simulink model "hexacopter_sim"  (R2023a)
settings: Solver=VariableStepAuto  StartTime=0.0  StopTime=15  MaxStep=0.001  RelTol=1e-7  EnableMultiTasking=on
values from neighbouring files (symbols this model uses):
  arm_length = 0.35    [hexacopter.m]    (also in hexacopter_unmodified.m)
  batteryDistanceFromCOG = -0.1    [hexacopter.m]    (also in hexacopter_unmodified.m)
  batteryMass = 0.56*2    (= 1.12)    [hexacopter.m]    (also in hexacopter_unmodified.m)
  batVolt = 3.7*cells    (= 14.8)    [hexacopter.m]    (also in hexacopter_unmodified.m)
  bodyMass = 1.2    [hexacopter.m]    (also in hexacopter_unmodified.m)
  deadCurrent = 0.3    [hexacopter.m]    (also in hexacopter_unmodified.m)
  droneMass = bodyMass + motorCount*(motorMass + propellerMassRaw)    (= 2.424)    [hexacopter.m]    (also in hexacopter_unmodified.m)
  h1al = 0.07    [discrete_controller_tuning.m]    (also in height_controller.m; hexacopter.m; hexacopter_unmodified.m)
  h1kp = 60    [hexacopter.m]    (also in hexacopter_unmodified.m)
  h1td = 1 / (sqrt(h1al) * target)    [height_controller.m]    (also in hexacopter.m = 1; hexacopter_unmodified.m = 1)
  h1ti = h1Ni * (1/ target)    (= 1.27118644068)    [height_controller.m]    (also in hexacopter.m = 1; hexacopter_unmodified.m = 1)
  h1val = 0.6    [discrete_controller_tuning.m]    (also in hexacopter.m = 0)
  h1vkp = 1    [hexacopter.m]
  h1vtd = 0    [hexacopter.m]
  h1vti = 1    [hexacopter.m]
  h_beta = 5    [hexacopter.m]    (also in hexacopter_unmodified.m)
  h_tau = 1.5    [hexacopter.m]    (also in hexacopter_unmodified.m)
  hoverControl = hoverVoltage/batVolt*1024    [hexacopter.m]    (also in hexacopter_unmodified.m)
  hoverVoltage = hoverCurrent * Ra + hoverRPM / Kv    [hexacopter.m]    (also in hexacopter_unmodified.m)
  KDrag = 1.5e-9    (= 1.5e-09)    [hexacopter.m]    (also in hexacopter_unmodified.m)
  Km = 60/(Kv * 2 * pi)    (= 0.013641852265)    [hexacopter.m]    (also in hexacopter_unmodified.m)
  Ktrust = 2.7e-5    (= 2.7e-05)    [hexacopter.m]    (also in hexacopter_unmodified.m)
  minimumMotorVolt = 1.0    (= 1)    [hexacopter.m]    (also in hexacopter_unmodified.m)
  motorMass = motorOnlyMass + 0.085    (= 0.187)    [hexacopter.m]    (also in hexacopter_unmodified.m)
  N = solve(eqn,V)    [temp.m]
  paal = 0.2    [hexacopter.m]    (also in hexacopter_unmodified.m)
  pakp = 0    [hexacopter.m]    (also in hexacopter_unmodified.m)
  pal = 0.5    [hexacopter.m]    (also in hexacopter_unmodified.m)
  patd = 1    [hexacopter.m]    (also in hexacopter_unmodified.m)
  pati = 100    [hexacopter.m]    (also in hexacopter_unmodified.m)
  pkp = 0    [hexacopter.m]    (also in hexacopter_unmodified.m)
  propellerMass = propellerMassRaw + 3*motorInertia/propellerRadius^2    (= 0.0220980494455)    [hexacopter.m]    (also in hexacopter_unmodified.m)
  ptd = 1    [hexacopter.m]    (also in hexacopter_unmodified.m)
  pti = 1    [hexacopter.m]    (also in hexacopter_unmodified.m)
  pushEnabled = 0    [hexacopter.m]    (also in hexacopter_unmodified.m)
  Ra = 0.083    [hexacopter.m]    (also in hexacopter_unmodified.m)
  raal = 0.2    [hexacopter.m]    (also in hexacopter_unmodified.m)
  rakp = 0    [hexacopter.m]    (also in hexacopter_unmodified.m)
  ral = 0.5    [hexacopter.m]    (also in hexacopter_unmodified.m)
  ratd = 1    [hexacopter.m]    (also in hexacopter_unmodified.m)
  rati = 100    [hexacopter.m]    (also in hexacopter_unmodified.m)
  rkp = 0    [hexacopter.m]    (also in hexacopter_unmodified.m)
  roll_limit = 10    [hexacopter.m]    (also in hexacopter_unmodified.m)
  rtd = 1    [hexacopter.m]    (also in hexacopter_unmodified.m)
  rti = 1    [hexacopter.m]    (also in hexacopter_unmodified.m)
  xal = 0.2    [hexacopter.m]    (also in hexacopter_unmodified.m = 1)
  xkp = 0    [hexacopter.m]    (also in hexacopter_unmodified.m)
  xtd = 1    [hexacopter.m]    (also in hexacopter_unmodified.m)
  xti = 100    [hexacopter.m]    (also in hexacopter_unmodified.m)
  xval = 0.2    [hexacopter.m]    (also in hexacopter_unmodified.m = 0.3; vel_controller.m = 0.3)
  xvkp = 0    [hexacopter.m]    (also in hexacopter_unmodified.m; vel_controller.m = 0.184077200147)
  xvtd = 1    [hexacopter.m]    (also in hexacopter_unmodified.m; vel_controller.m = 1 / (sqrt(xval) * target))
  xvti = 100    [hexacopter.m]    (also in hexacopter_unmodified.m; vel_controller.m = 0)
  yaal = 0.5    [hexacopter.m]    (also in hexacopter_unmodified.m)
  yakp = 0    [hexacopter.m]    (also in hexacopter_unmodified.m)
  yal = 0.5    [hexacopter.m]    (also in hexacopter_unmodified.m)
  yatd = 1    [hexacopter.m]    (also in hexacopter_unmodified.m)
  yati = 100    [hexacopter.m]    (also in hexacopter_unmodified.m)
  yaw_limit = 45    [hexacopter.m]    (also in hexacopter_unmodified.m)
  yiLim = 500    [hexacopter.m]    (also in hexacopter_unmodified.m)
  ykp = 0    [hexacopter.m]    (also in hexacopter_unmodified.m)
  ytd = 0    [hexacopter.m]    (also in hexacopter_unmodified.m)
  yti = 1000    [hexacopter.m]    (also in hexacopter_unmodified.m)
  yval = 0.3    [hexacopter.m]    (also in hexacopter_unmodified.m)
  yvkp = 0    [hexacopter.m]    (also in hexacopter_unmodified.m)
  yvtd = 1    [hexacopter.m]    (also in hexacopter_unmodified.m)
  yvti = 100    [hexacopter.m]    (also in hexacopter_unmodified.m)
undefined symbols (not defined in the file or in its folder): h2al, h2kp, h2td, h2ti, X, Y, Z
libraries: sm_lib x52, nesl_utility x34, simulink x3
(part 1 of 3)
settings Model: Creator=chr  LastModifiedBy=marcu
settings SolverCC: AlgebraicLoopSolver=TrustRegion
settings DataIOCC: LimitDataPoints=on  SaveFormat=Array  ReturnWorkspaceOutputs=off
settings OptimizationCC: LifeSpan=inf
settings DebuggingCC: UnconnectedInputMsg=warning  UnconnectedOutputMsg=warning  UnconnectedLineMsg=warning  SFUnexpectedBacktrackingDiag=warning  SFNoUnconditionalDefaultTransitionDiag=warning  SFExecutionAtInitializationDiag=none  ArithmeticOperatorsInVariantConditions=warning
settings HardwareCC: ProdBitPerPointer=32  ProdBitPerSizeT=32  ProdBitPerPtrDiffT=32  ProdLargestAtomicFloat=None  ProdIntDivRoundTo=Undefined  ProdEndianess=Unspecified  ProdWordSize=32  ProdHWDeviceType=32-bit Generic
settings ModelReferenceCC: EnableRefExpFcnMdlSchedulingChecks=on  PropagateSignalLabelsOutOfModel=off
settings SFSimCC: SimUseLocalCustomCode=off  CustomCodeUndefinedFunction=UseInterfaceOnly
settings RTWCC: RTWUseLocalCustomCode=off  DLArmComputeVersion=19.05
settings CodeAppCC: StateflowObjectComments=on
settings GRTTargetCC: TargetLangStandard=C89/C90 (ANSI)
settings ConfigComp: CovMetricSettings=dw  CovSaveCumulativeToWorkspaceVar=on  CovSaveSingleToWorkspaceVar=on  CovExternalEMLEnable=off
settings SimscapeCC: SimscapeNormalizeSystem=off  SimscapeLogType=all  SimscapeLogDataHistory=10000
settings ConfigurationSet: Description=SimMechanics 2G

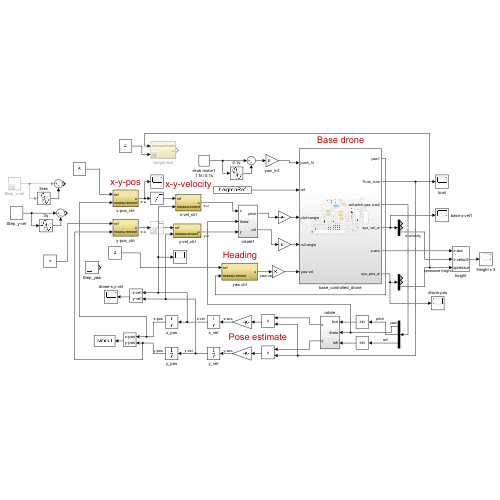
[thumbnail: Simulink's stored preview of the top-level diagram]
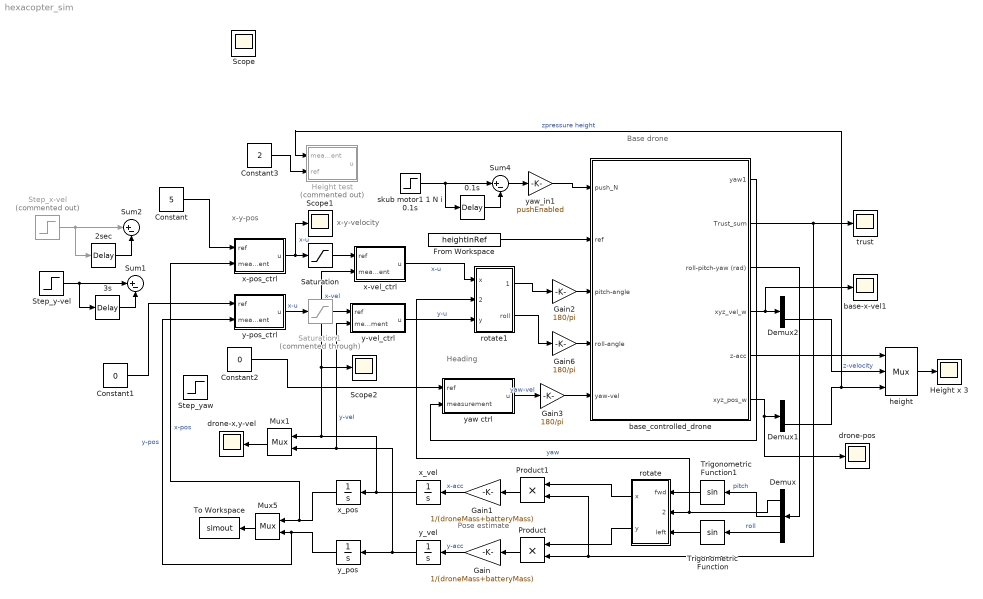
== system hexacopter_sim ==
  note: x-y-velocity
  note: Heading
  note: Pose estimate
  note: Base drone
  note: x-y-pos
  0.1s : TransportDelay  DelayTime=0.1
  2sec : TransportDelay  DelayTime=2
  3s : TransportDelay  DelayTime=2
  Constant : Constant  Value=5
  Constant1 : Constant  Value=0
  Constant2 : Constant  Value=0
  Constant3 : Constant  Value=2
  Demux : Demux  Outputs=3
  Demux1 : Demux  Outputs=3
  Demux2 : Demux  Outputs=3
  From Workspace : FromWorkspace  VariableName=heightInRef
  Gain : Gain  Gain=1/(droneMass+batteryMass)
  Gain1 : Gain  Gain=1/(droneMass+batteryMass)
  Gain2 : Gain  Gain=180/pi
  Gain3 : Gain  Gain=180/pi
  Gain6 : Gain  Gain=180/pi
  Height test : Subsystem  Commented=on
  Height x 3 : Scope
  Mux1 : Mux  Inputs=2
      settings: DisplayOption=signals
  Mux5 : Mux  Inputs=2
      settings: DisplayOption=signals
  Product : Product
  Product1 : Product
  Saturation : Saturate  UpperLimit=1  LowerLimit=-1
  Saturation1 : Saturate  Commented=through  UpperLimit=1  LowerLimit=-1
  Scope1 : Scope
  Scope2 : Scope
  Step_x-vel : Step  Commented=on  Time=5  After=0.1  SampleTime=0
  Step_y-vel : Step  Time=3  After=4  SampleTime=0
  Step_yaw : Step  Time=3.0  After=pi/2  SampleTime=0
  Sum1 : Sum  Inputs=|+-
  Sum2 : Sum  Inputs=|+-
  Sum4 : Sum  Inputs=|+-
  To Workspace : ToWorkspace  VariableName=simout  SaveFormat=Timeseries  SampleTime=-1
  Trigonometric Function : Trigonometry
  Trigonometric Function1 : Trigonometry
  base-x-vel1 : Scope
  base_controlled_drone : Subsystem
  drone-pos : Scope
  drone-x,y-vel : Scope
  height : Mux  Inputs=3
      settings: DisplayOption=signals
  rotate : Subsystem
  rotate1 : Subsystem
  skub motor1 1 N i 0.1s : Step  Time=2  After=4  SampleTime=0
  trust : Scope
  x-pos_ctrl : Subsystem
  x-vel_ctrl : Subsystem
  x_pos : Integrator
  x_vel : Integrator
  y-pos_ctrl : Subsystem
  y-vel_ctrl : Subsystem
  y_pos : Integrator
  y_vel : Integrator
  yaw ctrl : Subsystem
  yaw_in1 : Gain  Gain=pushEnabled
  Scope : Scope
  wires:
  Product/1 -> Gain/1
  Gain/1 -> y_vel/1  "y-acc"
  y_vel/1 -> y_pos/1, Mux1/2, y-vel_ctrl/2(measurement)  "y-vel"
  x_vel/1 -> x_pos/1, Mux1/1, x-vel_ctrl/2(measurement), Scope2/1  "x-vel"
  Gain1/1 -> x_vel/1  "x-acc"
  Product1/1 -> Gain1/1
  Mux1/1 -> drone-x,y-vel/1
  Mux5/1 -> To Workspace/1
  x_pos/1 -> x-pos_ctrl/2(measurement), Mux5/1  "x-pos"
  y_pos/1 -> y-pos_ctrl/2(measurement), Mux5/2  "y-pos"
  base_controlled_drone/5(z-acc) -> height/1
  base_controlled_drone/2(Trust_sum) -> trust/1, Product1/2, Product/2
  Demux1/3 -> Height test/1(measurement), height/3  "zpressure height"
  yaw ctrl/1(u) -> Gain3/1  "yaw-vel"
  base_controlled_drone/1(yaw1) -> yaw ctrl/2(measurement)
  base_controlled_drone/3(roll-pitch-yaw (rad)) -> Demux/1
  base_controlled_drone/4(xyz_vel_w) -> base-x-vel1/1, Demux2/1
  base_controlled_drone/6(xyz_pos_w) -> Demux1/1, drone-pos/1
  Demux2/3 -> height/2  "z-velocity"
  Demux/3 -> Trigonometric Function/1  "roll"
  Demux/2 -> Trigonometric Function1/1  "pitch"
  0.1s/1 -> Sum4/2
  skub motor1 1 N i 0.1s/1 -> 0.1s/1, Sum4/1
  Sum4/1 -> yaw_in1/1
  yaw_in1/1 -> base_controlled_drone/1(push_N)
  Step_y-vel/1 -> 3s/1, Sum1/1
  3s/1 -> Sum1/2
  2sec/1 -> Sum2/2
  Step_x-vel/1 -> 2sec/1, Sum2/1
  y-vel_ctrl/1(u) -> rotate1/3(y)  "y-u"
  Trigonometric Function1/1 -> rotate/1(fwd)
  Demux/1 -> rotate1/2(theta), rotate/2(theta)  "yaw"
  Trigonometric Function/1 -> rotate/3(left)
  rotate/1(x) -> Product1/1
  rotate/2(y) -> Product/1
  x-vel_ctrl/1(u) -> rotate1/1(x)  "x-u"
  rotate1/1(pitch) -> Gain2/1
  rotate1/2(roll) -> Gain6/1
  Gain6/1 -> base_controlled_drone/4(roll-angle)
  Gain2/1 -> base_controlled_drone/3(pitch-angle)
  Gain3/1 -> base_controlled_drone/5(yaw-vel)
  Constant1/1 -> y-pos_ctrl/1(ref)
  Constant/1 -> x-pos_ctrl/1(ref)
  x-pos_ctrl/1(u) -> Scope1/1, Saturation/1  "x-u"
  y-pos_ctrl/1(u) -> Saturation1/1  "x-u"
  Constant2/1 -> yaw ctrl/1(ref)
  Constant3/1 -> Height test/2(ref)
  Saturation1/1 -> y-vel_ctrl/1(ref)
  Saturation/1 -> x-vel_ctrl/1(ref)
  From Workspace/1 -> base_controlled_drone/2(ref)
  height/1 -> Height x 3/1

== system hexacopter_sim/Height test ==
  measurement : Inport
  ref : Inport  Port=2
  Constant : Constant  Value=hoverControl
  Gain : Gain  Gain=h2kp
  Gain1 : Gain  Gain=1/h2ti
  Gain2 : Gain  Gain=1/102.4
  Integrator : Integrator  InitialCondition=hoverVoltage  LimitOutput=on  UpperSaturationLimit=batVolt  LowerSaturationLimit=-batVolt
  Sum : Sum  Inputs=|+-
  Sum1 : Sum  Inputs=+++
  Transfer Fcn : TransferFcn  Numerator=[h2td 1]  Denominator=[h2al*h2td 1]
  u : Outport  VectorParamsAs1DForOutWhenUnconnected=off
  wires:
  ref/1 -> Sum/1
  measurement/1 -> Transfer Fcn/1
  Transfer Fcn/1 -> Sum/2
  Sum/1 -> Gain/1
  Integrator/1 -> Sum1/2
  Gain/1 -> Sum1/3, Gain1/1
  Gain1/1 -> Integrator/1
  Sum1/1 -> u/1
  Constant/1 -> Gain2/1
  Gain2/1 -> Sum1/1

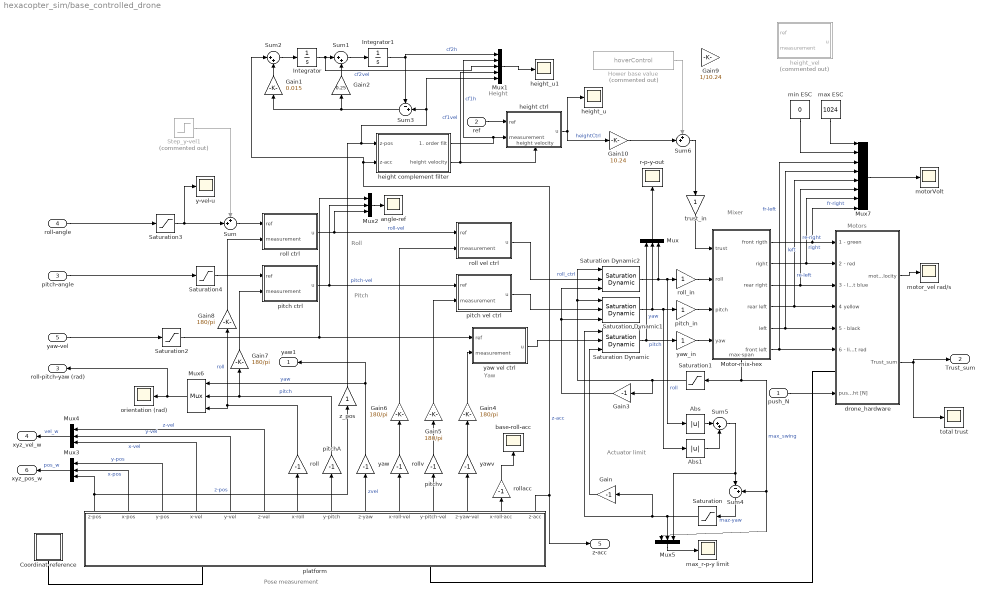
== system hexacopter_sim/base_controlled_drone ==
  note: Height
  note: Roll
  note: Pitch
  note: Yaw
  note: Mixer
  note: Motors
  note: Pose measurement
  note: Actuator
      | limit
  push_N : Inport
  ref : Inport  Port=2
  pitch-angle : Inport  Port=3
  roll-angle : Inport  Port=4
  yaw-vel : Inport  Port=5
  Abs : Abs  SaturateOnIntegerOverflow=off
  Abs1 : Abs  SaturateOnIntegerOverflow=off
  Coordinat-reference : Subsystem
  Gain : Gain  Gain=-1
  Gain1 : Gain  Gain=0.015
  Gain10 : Gain  Gain=10.24
  Gain2 : Gain  Gain=0.25
  Gain3 : Gain  Gain=-1
  Gain{4..8} (5 alike) : Gain  Gain=180/pi
  Gain9 : Gain  Gain=1/10.24
  Hower base value : Constant  Commented=on  Value=hoverControl
  Integrator : Integrator
  Integrator1 : Integrator
  Motor-mix-hex : Subsystem
      settings: PortSchema="{\"entries\":[{\"content\":{\"sides\":[{\"content\":{\"connectorIds\":[\"In1\",\"In2\",\"In3\",\"In4\"]},\"type\":\"ConnectorPlacement.EquallySpacedRectSide\",\"uuid\":\"306a341c-ac5f-471d-a132-016b70a80876\"},{\"content\":{\"connectorIds\":[\"Out1\",\"Out2\",\"Out3\",\"Out4\",\"Out5\",\"Out6\"],\"side\":\"RIGHT\"},\"type\":\"ConnectorPlacement.EquallySpacedRectSide\",\"uuid\":\"ef186704-dd28-4c65-8a41-6a93d20ba170\"},{\"content\":{\"connectorIds\":[],\"side\":\"TOP\"},\"type\":\"ConnectorPlacement.EquallySpacedRectSide\",\"uuid\":\"97573a1a-e480-4bb7-b791-daec4a837e10\"},{\"content\":{\"connectorIds\":[\"Out7\"],\"side\":\"BOTTOM\"},\"type\":\"ConnectorPlacement.EquallySpacedRectSide\",\"uuid\":\"e76c5da7-f0c9-4cfe-962d-1d4a2d2f611a\"}]},\"type\":\"ConnectorPlacement.EquallySpacedConnector\",\"uuid\":\"3cd8fd48-1c03-4a94-b99a-acef471dd5f6\"}],\"packageUris\":[\"http://schema.mathworks.com/mf0/Connector/19700101\"],\"version\":\"1.0\"}"
  Mux{,2..6} (6 alike) : Mux  Inputs=3
      Mux6 settings: DisplayOption=signals
  Mux1 : Mux  Inputs=5
  Mux7 : Mux  Inputs=8
  Saturation : Saturate  UpperLimit=500  LowerLimit=50
  Saturation Dynamic : simulink/Discontinuities/Saturation Dynamic  OutMin=[]  OutMax=[]  OutDataTypeStr=Inherit: Same as second input  OutDataType=fixdt(1, 16)  OutScaling=2^-10  DoSatur=off
  Saturation Dynamic1 : simulink/Discontinuities/Saturation Dynamic  OutMin=[]  OutMax=[]  OutDataTypeStr=Inherit: Same as second input  OutDataType=fixdt(1, 16)  OutScaling=2^-10  DoSatur=off
  Saturation Dynamic2 : simulink/Discontinuities/Saturation Dynamic  OutMin=[]  OutMax=[]  OutDataTypeStr=Inherit: Same as second input  OutDataType=fixdt(1, 16)  OutScaling=2^-10  DoSatur=off
  Saturation1 : Saturate  UpperLimit=250  LowerLimit=50
  Saturation2 : Saturate  UpperLimit=yaw_limit  LowerLimit=-yaw_limit
  Saturation3 : Saturate  UpperLimit=roll_limit  LowerLimit=-roll_limit
  Saturation4 : Saturate  UpperLimit=roll_limit  LowerLimit=-roll_limit
  Step_y-vel1 : Step  Commented=on  Time=5  After=0.03  SampleTime=0
  Sum : Sum  Inputs=++|
  Sum1 : Sum  Inputs=|++
  Sum2 : Sum  Inputs=|++
  Sum3 : Sum  Inputs=-+|
  Sum4 : Sum  Inputs=|-+
  Sum5 : Sum  Inputs=|++
  Sum6 : Sum  Inputs=++|
  angle-ref : Scope
  base-roll-acc : Scope
  drone_hardware : Subsystem
      settings: PortSchema="{\"entries\":[{\"content\":{\"sides\":[{\"content\":{\"connectorIds\":[\"In1\",\"In2\",\"In3\",\"In4\",\"In5\",\"In6\",\"LConn1\",\"In7\"]},\"type\":\"ConnectorPlacement.EquallySpacedRectSide\",\"uuid\":\"51e20491-184f-4c13-ad67-858d0ecfecfd\"},{\"content\":{\"connectorIds\":[\"Out1\",\"Out2\"],\"side\":\"RIGHT\"},\"type\":\"ConnectorPlacement.EquallySpacedRectSide\",\"uuid\":\"dd38fec1-9b5b-4065-9c26-bdf68d278980\"},{\"content\":{\"connectorIds\":[],\"side\":\"TOP\"},\"type\":\"ConnectorPlacement.EquallySpacedRectSide\",\"uuid\":\"f644b8cb-3aa9-4068-acaf-6a442e3f1948\"}]},\"type\":\"ConnectorPlacement.EquallySpacedConnector\",\"uuid\":\"e398b018-d970-47a6-aa8b-d81f44328f20\"}],\"packageUris\":[\"http://schema.mathworks.com/mf0/Connector/19700101\"],\"version\":\"1.0\"}"
  height complement filter : Subsystem
  height ctrl : Subsystem
      settings: PortSchema="{\"entries\":[{\"content\":{\"sides\":[{\"content\":{\"connectorIds\":[\"In1\",\"In2\"]},\"type\":\"ConnectorPlacement.EquallySpacedRectSide\",\"uuid\":\"271a1acb-e3e8-4cfb-9f31-dd4cafd2265e\"},{\"content\":{\"connectorIds\":[\"Out1\"],\"side\":\"RIGHT\"},\"type\":\"ConnectorPlacement.EquallySpacedRectSide\",\"uuid\":\"68f874e9-90a1-4368-8575-5a82b085067c\"},{\"content\":{\"connectorIds\":[],\"side\":\"TOP\"},\"type\":\"ConnectorPlacement.EquallySpacedRectSide\",\"uuid\":\"569a036c-ce5f-4131-b1de-fc83d9f7b4fb\"},{\"content\":{\"connectorIds\":[\"In3\"],\"side\":\"BOTTOM\"},\"type\":\"ConnectorPlacement.EquallySpacedRectSide\",\"uuid\":\"21cdb078-780e-47a7-9ed6-f7bdbb9c6310\"}]},\"type\":\"ConnectorPlacement.EquallySpacedConnector\",\"uuid\":\"571821a6-3ef7-4905-96ac-3b6dbf9c7847\"}],\"packageUris\":[\"http://schema.mathworks.com/mf0/Connector/19700101\"],\"version\":\"1.0\"}"
  height_u : Scope
  height_u1 : Scope
  height_vel : Subsystem  Commented=on
  max ESC : Constant  Value=1024
  max_r-p-y limit : Scope
  min ESC : Constant  Value=0
  motorVolt : Scope
  motor_vel rad/s : Scope
  orientation (rad) : Scope
  pitch ctrl : Subsystem
  pitch vel ctrl : Subsystem
  pitchA : Gain  Gain=-1
  pitch_in : Gain
  pitchv : Gain  Gain=-1
  platform : Subsystem
  r-p-y-out : Scope
  roll : Gain  Gain=-1
  roll ctrl : Subsystem
  roll vel ctrl : Subsystem
  roll_in : Gain
  rollacc : Gain  Gain=-1
  rollv : Gain  Gain=-1
  total trust : Scope
  trust_in : Gain
  y-vel-u : Scope
  yaw : Gain  Gain=-1
  yaw vel ctrl : Subsystem
  yaw_in : Gain
  yawv : Gain  Gain=-1
  z_pos : Gain
  yaw1 : Outport
  Trust_sum : Outport  Port=2
  roll-pitch-yaw (rad) : Outport  Port=3
  xyz_vel_w : Outport  Port=4
  z-acc : Outport  Port=5
  xyz_pos_w : Outport  Port=6
  wires:
  Mux7/1 -> motorVolt/1
  Saturation Dynamic1/1 -> Mux/2, Abs1/1, pitch_in/1  "pitch"
  platform/3(y-pos) -> Mux3/1  "y-pos"
  drone_hardware/1(motor_velocity) -> motor_vel rad/s/1
  rollv/1 -> Gain6/1
  platform/4(x-vel) -> Mux4/3  "x-vel"
  platform/8(y-pitch) -> pitchA/1
  platform/2(x-pos) -> Mux3/2  "x-pos"
  pitch_in/1 -> Motor-mix-hex/3(pitch)
  Mux2/1 -> angle-ref/1
  Step_y-vel1/1 -> Sum/1
  platform/7(x-roll) -> roll/1
  pitch ctrl/1(u) -> Mux2/2, pitch vel ctrl/1(ref)  "pitch-vel"
  rollacc/1 -> base-roll-acc/1
  Motor-mix-hex/2(right) -> Mux7/7, drone_hardware/2(2 - red)  "right"
  Saturation Dynamic2/1 -> Mux/3, Abs/1, roll_in/1  "roll"
  Sum/1 -> roll ctrl/1(ref)
  platform/14(z-acc) -> Sum2/1, height complement filter/2(z-acc), z-acc/1  "z-acc"
  Saturation4/1 -> pitch ctrl/1(ref)
  platform/11(y-pitch-vel) -> pitchv/1
  min ESC/1 -> Mux7/2
  Mux6/1 -> roll-pitch-yaw (rad)/1, orientation (rad)/1
  Mux3/1 -> xyz_pos_w/1  "pos_w"
  Motor-mix-hex/1(front rigth) -> Mux7/8, drone_hardware/1(1 - green)  "fr-right"
  yaw/1 -> yaw1/1, Mux6/1  "yaw"
  platform/13(x-roll-acc) -> rollacc/1
  drone_hardware/2(Trust_sum) -> Trust_sum/1, total trust/1
  platform/9(z-yaw) -> yaw/1  "zvel"
  platform/10(x-roll-vel) -> rollv/1
  pitchv/1 -> Gain5/1
  Motor-mix-hex/4(rear left) -> Mux7/5, drone_hardware/4(4 yellow)  "re-left"
  Motor-mix-hex/6(front left) -> Mux7/3, drone_hardware/6(6 - light red)  "fr-left"
  Saturation Dynamic/1 -> Mux/1, yaw_in/1  "yaw"
  max ESC/1 -> Mux7/1
  Saturation3/1 -> y-vel-u/1, Sum/2
  platform/5(y-vel) -> Mux4/2  "y-vel"
  roll ctrl/1(u) -> Mux2/3, roll vel ctrl/1(ref)  "roll-vel"
  Mux/1 -> r-p-y-out/1
  platform/1(z-pos) -> z_pos/1, Mux3/3  "z-pos"
  Mux4/1 -> xyz_vel_w/1  "vel_w"
  pitchA/1 -> Gain7/1, Mux6/2  "pitch"
  push_N/1 -> drone_hardware/7(push right [N])
  platform/6(z-vel) -> Mux4/1  "z-vel"
  height ctrl/1(u) -> Gain10/1, height_u/1  "heightCtrl"
  Motor-mix-hex/3(rear right) -> Mux7/6, drone_hardware/3(3 - light blue)  "re-right"
  platform/12(z-yaw-vel) -> yawv/1
  Motor-mix-hex/5(left) -> Mux7/4, drone_hardware/5(5 - black)  "left"
  yaw_in/1 -> Motor-mix-hex/4(yaw)
  roll_in/1 -> Motor-mix-hex/2(roll)
  roll/1 -> Gain8/1, Mux6/3  "roll"
  trust_in/1 -> Motor-mix-hex/1(trust)
  height complement filter/1(1. order filt) -> Mux1/2, height ctrl/2(measurement)  "cf1h"
  yaw vel ctrl/1(u) -> Saturation Dynamic/2
  pitch vel ctrl/1(u) -> Saturation Dynamic1/2
  roll vel ctrl/1(u) -> Saturation Dynamic2/2  "roll_ctrl"
  Gain/1 -> Saturation Dynamic/3
  height complement filter/2(height velocity) -> Mux1/4, height ctrl/3(height velocity)  "cf1vel"
  Gain1/1 -> Sum2/2
  Gain2/1 -> Sum1/2
  Sum3/1 -> Gain1/1, Gain2/1
  Integrator1/1 -> Sum3/1, Mux1/1  "cf2h"
  Sum2/1 -> Integrator/1
  Integrator/1 -> Mux1/3, Sum1/1  "cf2vel"
  Sum1/1 -> Integrator1/1
  Mux1/1 -> height_u1/1
  Motor-mix-hex/7(max-span) -> Saturation1/1, Sum4/2, Mux5/1  "max_swing"
  Sum4/1 -> Saturation/1  "maz-yaw"
  Abs/1 -> Sum5/1
  Abs1/1 -> Sum5/2
  Gain3/1 -> Saturation Dynamic1/3, Saturation Dynamic2/3
  Mux5/1 -> max_r-p-y limit/1
  Sum5/1 -> Mux5/3, Sum4/1
  Saturation/1 -> Gain/1, Saturation Dynamic/1, Mux5/2
  Saturation1/1 -> Saturation Dynamic1/1, Saturation Dynamic2/1, Gain3/1
  yawv/1 -> Gain4/1
  Gain4/1 -> yaw vel ctrl/2(measurement)
  Gain5/1 -> pitch vel ctrl/2(measurement)
  Gain6/1 -> roll vel ctrl/2(measurement)
  Gain7/1 -> pitch ctrl/2(measurement)
  Gain8/1 -> roll ctrl/2(measurement)
  Saturation2/1 -> Mux2/1, yaw vel ctrl/1(ref)
  roll-angle/1 -> Saturation3/1
  yaw-vel/1 -> Saturation2/1
  pitch-angle/1 -> Saturation4/1
  ref/1 -> height ctrl/1(ref)
  Sum6/1 -> trust_in/1
  Hower base value/1 -> Sum6/1
  ? -> height_vel/1(ref)
  z_pos/1 -> Mux1/5, Sum3/2, height complement filter/1(z-pos)
  Gain10/1 -> Sum6/2
  connections:
  platform/LConn2 -- drone_hardware/LConn1
  platform/LConn1 -- Coordinat-reference/RConn1

== system hexacopter_sim/rotate ==
  fwd : Inport
  theta : Inport  Port=2
  left : Inport  Port=3
  Cos : Trigonometry  Operator=cos
  Product{2..5} (4 alike) : Product
  Sum : Sum  Inputs=|++
  Sum3 : Sum  Inputs=|-+
  Trigonometric Function2 : Trigonometry
  x : Outport
  y : Outport  Port=2
  wires:
  theta/1 -> Cos/1, Trigonometric Function2/1  "yaw"
  Sum/1 -> x/1
  Product3/1 -> Sum3/2
  Product4/1 -> Sum/2
  Trigonometric Function2/1 -> Product5/2, Product4/1  "sin"
  left/1 -> Product4/2, Product3/2
  Sum3/1 -> y/1
  fwd/1 -> Product5/1, Product2/1
  Product2/1 -> Sum/1
  Cos/1 -> Product3/1, Product2/2  "cos"
  Product5/1 -> Sum3/1

== system hexacopter_sim/rotate1 ==
  x : Inport
  theta : Inport  Port=2
  y : Inport  Port=3
  Cos : Trigonometry  Operator=cos
  Product{2..5} (4 alike) : Product
  Sum : Sum  Inputs=|+-
  Sum3 : Sum  Inputs=|++
  Trigonometric Function2 : Trigonometry
  pitch : Outport
  roll : Outport  Port=2
  wires:
  Product5/1 -> Sum3/1
  Cos/1 -> Product2/2, Product3/1  "cos"
  Product2/1 -> Sum/1
  x/1 -> Product2/1, Product5/1
  Sum3/1 -> roll/1
  y/1 -> Product3/2, Product4/2
  Trigonometric Function2/1 -> Product4/1, Product5/2  "sin"
  Product4/1 -> Sum/2
  Product3/1 -> Sum3/2
  Sum/1 -> pitch/1
  theta/1 -> Trigonometric Function2/1, Cos/1  "yaw"

== system hexacopter_sim/x-pos_ctrl ==
  ref : Inport
  measurement : Inport  Port=2
  Gain : Gain  Gain=xkp
  Gain1 : Gain  Commented=on  Gain=1/xti
  Integrator : Integrator  Commented=on
  Sum : Sum  Inputs=|+-
  Sum1 : Sum  Inputs=|++
  Transfer Fcn : TransferFcn  Commented=through  Numerator=[xtd 1]  Denominator=[xal*xtd 1]
  u : Outport  VectorParamsAs1DForOutWhenUnconnected=off
  wires:
  ref/1 -> Sum/1
  measurement/1 -> Transfer Fcn/1
  Transfer Fcn/1 -> Sum/2
  Sum/1 -> Gain/1
  Gain1/1 -> Integrator/1
  Gain/1 -> Gain1/1, Sum1/2
  Sum1/1 -> u/1
  Integrator/1 -> Sum1/1

== system hexacopter_sim/x-vel_ctrl ==
  ref : Inport
  measurement : Inport  Port=2
  Gain : Gain  Gain=xvkp
  Gain1 : Gain  Gain=1/xvti
  Integrator : Integrator  LimitOutput=on  UpperSaturationLimit=1  LowerSaturationLimit=-1
  Sum : Sum  Inputs=|+-
  Sum1 : Sum  Inputs=|++
  Transfer Fcn : TransferFcn  Numerator=[xvtd 1]  Denominator=[xval*xvtd 1]
  u : Outport  VectorParamsAs1DForOutWhenUnconnected=off
  wires:
  ref/1 -> Sum/1
  measurement/1 -> Transfer Fcn/1
  Transfer Fcn/1 -> Sum/2
  Sum/1 -> Gain/1
  Integrator/1 -> Sum1/1
  Gain/1 -> Gain1/1, Sum1/2
  Gain1/1 -> Integrator/1
  Sum1/1 -> u/1

== system hexacopter_sim/y-pos_ctrl ==
  ref : Inport
  measurement : Inport  Port=2
  Gain : Gain  Gain=xkp
  Gain1 : Gain  Commented=on  Gain=1/xti
  Integrator : Integrator  Commented=on
  Sum : Sum  Inputs=|+-
  Sum1 : Sum  Inputs=|++
  Transfer Fcn : TransferFcn  Numerator=[xtd 1]  Denominator=[xal*xtd 1]
  u : Outport  VectorParamsAs1DForOutWhenUnconnected=off
  wires:
  ref/1 -> Sum/1
  measurement/1 -> Transfer Fcn/1
  Transfer Fcn/1 -> Sum/2
  Sum/1 -> Gain/1
  Gain1/1 -> Integrator/1
  Gain/1 -> Gain1/1, Sum1/2
  Sum1/1 -> u/1
  Integrator/1 -> Sum1/1

== system hexacopter_sim/y-vel_ctrl ==
  ref : Inport
  measurement : Inport  Port=2
  Gain : Gain  Gain=yvkp
  Gain1 : Gain  Commented=on  Gain=1/yvti
  Integrator : Integrator  Commented=on  InitialCondition=hoverVoltage  LimitOutput=on  UpperSaturationLimit=batVolt  LowerSaturationLimit=-batVolt
  Sum : Sum  Inputs=|+-
  Sum1 : Sum  Inputs=|++
  Transfer Fcn : TransferFcn  Numerator=[yvtd 1]  Denominator=[yval*yvtd 1]
  u : Outport  VectorParamsAs1DForOutWhenUnconnected=off
  wires:
  Gain1/1 -> Integrator/1
  Gain/1 -> Sum1/2, Gain1/1
  Integrator/1 -> Sum1/1
  Sum/1 -> Gain/1
  Transfer Fcn/1 -> Sum/2
  measurement/1 -> Transfer Fcn/1
  ref/1 -> Sum/1
  Sum1/1 -> u/1

== system hexacopter_sim/yaw ctrl ==
  ref : Inport
  measurement : Inport  Port=2
  Gain : Gain  Gain=yakp
  Gain1 : Gain  Commented=on  Gain=1/yati
  Integrator : Integrator  Commented=on  InitialCondition=hoverVoltage  LimitOutput=on  UpperSaturationLimit=batVolt  LowerSaturationLimit=-batVolt
  Sum : Sum  Inputs=|+-
  Sum1 : Sum  Inputs=|++
  Transfer Fcn : TransferFcn  Commented=through  Numerator=[yatd 1]  Denominator=[yaal*yatd 1]
  Transfer Fcn1 : TransferFcn  Numerator=[yatd 1]  Denominator=[yaal*yatd 1]
  u : Outport  VectorParamsAs1DForOutWhenUnconnected=off
  wires:
  ref/1 -> Sum/1
  measurement/1 -> Transfer Fcn/1
  Transfer Fcn/1 -> Sum/2
  Sum/1 -> Gain/1
  Sum1/1 -> Transfer Fcn1/1
  Integrator/1 -> Sum1/1
  Gain/1 -> Gain1/1, Sum1/2
  Gain1/1 -> Integrator/1
  Transfer Fcn1/1 -> u/1

== system hexacopter_sim/base_controlled_drone/Coordinat-reference ==
  Mechanism Configuration : sm_lib/Utilities/Mechanism Configuration  UniformGravity=Constant  GravityVector=[0 0 -9.82]  GravityVectorUnits=m/s^2  LinearizationDelta=0.001  JointModeTransitionNonlinearIterations=2
  Solver Configuration : nesl_utility/Solver Configuration  PhysicalDomain=network_engine_domain  SubClassName=solver  LeftPortType=input  RightPortType=generic  Tones=[]  Harmonics=[]  SimulateNoise=off  Profile=off  UseLocalSampling=off  EnableSwitchedLinearOptims=on  FrequencyDomain=off  UseCCode=off  RelTol=0.001  AbsTol=1e-06  MinStep=1e-09  ToWorkspace=off  RevertToSquareIcSolve=off  NumHomotopyIterations=100  PhasorMode=off  PhasorModeNumHarmonics=1  ConsistencySolver=NEWTON_FTOL  IndexReductionMethod=DerivativeReplacement  DoDC=off  ResidualTolerance=1e-09  ConsistencyTolSource=GLOBAL  ConsistencyAbsTol=0.001  ConsistencyRelTol=0.001  ConsistencyTolFactor=0.001  UseLocalSolver=off  LocalSolverChoice=NE_BACKWARD_EULER_ADVANCER  ResolveIndetEquations=on  FunctionEvalNumThread=1  LocalSolverSampleTime=0.001  DoFixedCost=off  MaxNonlinIter=3  MaxModeIter=2  ComputeImpulses=off  ImpulseIterations=2  LinearAlgebra=Sparse  LinearAlgebraNumThread=0  EquationFormulation=NE_TIME_EF  DelaysMemoryBudget=1024  AutomaticFiltering=on  FilteringTimeConstant=0.001  PartitionStorageMethod=AS_NEEDED  PartitionMemoryBudget=1024  PartitionMethod=FAST
  World Frame : sm_lib/Frames and Transforms/World Frame
  ground : sm_lib/Body Elements/Brick Solid  GraphicAmbientColor=[0.15 0.15 0.15 1.0]  BasedOnType=Mass  BrickDimensions=[1 1 0.01]  BrickDimensionsUnits=m  CenterOfMass=[0 0 0]  CenterOfMassUnits=m  GraphicDiffuseColor=[0.2 0.5 0.2]  Density=1000  DensityUnits=kg/(m^3)  DoExposeReferenceFrame=on  GraphicEmissiveColor=[0.0 0.0 0.0 1.0]  ExportEntireGeometry=off  SerializedFrames=<Frames/>  MarkerShape=Sphere  MarkerSize=10  GraphicType=FromGeometry  InertiaType=CalculateFromGeometry  Mass=1  MassUnits=kg  MomentsOfInertia=[1 1 1]  MomentsOfInertiaUnits=kg*m^2  GraphicOpacity=1.0  ProductsOfInertia=[0 0 0]  ProductsOfInertiaUnits=kg*m^2  GraphicShininess=75  GraphicSpecularColor=[0.5 0.5 0.5 1.0]  GraphicVisPropType=SimpleVisualProperties
  Conn1 : PMIOPort  Side=Right
  connections:
  Solver Configuration/RConn1 -- Conn1/RConn1 -- ground/RConn1 -- World Frame/RConn1 -- Mechanism Configuration/RConn1

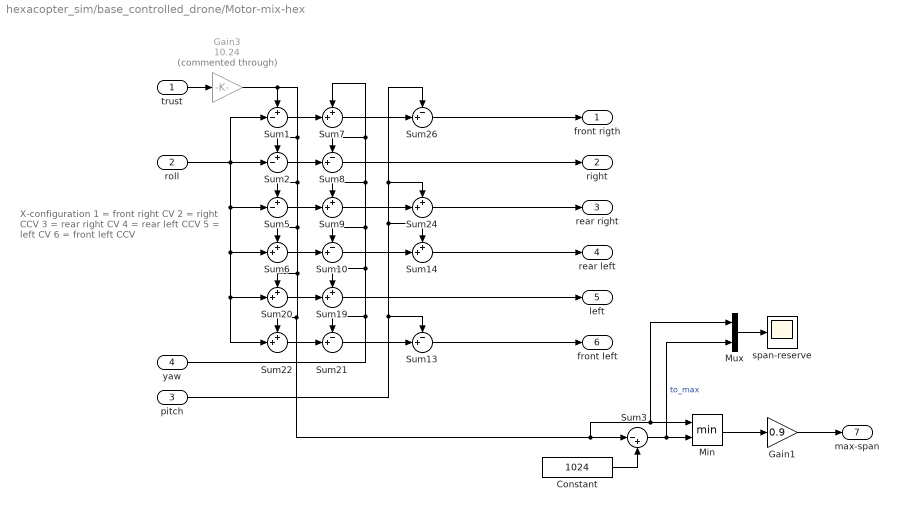
== system hexacopter_sim/base_controlled_drone/Motor-mix-hex ==
  note: X-configuration
      | 1 = front right CV
      | 2 = right        CCV
      | 3 = rear right CV
      | 4 = rear left   CCV
      | 5 = left          CV
      | 6 = front left CCV
  trust : Inport
  roll : Inport  Port=2
  pitch : Inport  Port=3
  yaw : Inport  Port=4
  Constant : Constant  Value=1024
  Gain1 : Gain  Gain=0.9
  Gain3 : Gain  Commented=through  Gain=10.24
  Min : MinMax  Inputs=2
  Mux : Mux  Inputs=2
  Sum1 : Sum  Inputs=+-|
  Sum{8,10,13,21,26} (5 alike) : Sum  Inputs=-+|
  Sum{6..7,9,14,19..20,22,24} (8 alike) : Sum  Inputs=++|
  Sum2 : Sum  Inputs=+-|
  Sum3 : Sum  Inputs=|-+
  Sum5 : Sum  Inputs=+-|
  span-reserve : Scope
  front rigth : Outport
  right : Outport  Port=2
  rear right : Outport  Port=3
  rear left : Outport  Port=4
  left : Outport  Port=5
  front left : Outport  Port=6
  max-span : Outport  Port=7
  wires:
  trust/1 -> Gain3/1
  Sum2/1 -> Sum8/2
  Sum22/1 -> Sum21/2
  Sum1/1 -> Sum7/2
  yaw/1 -> Sum21/1, Sum7/1, Sum8/1, Sum9/1, Sum10/1, Sum19/1
  Sum5/1 -> Sum9/2
  Sum21/1 -> Sum13/2
  Sum6/1 -> Sum10/2
  Sum7/1 -> Sum26/2
  Sum9/1 -> Sum24/2
  Sum20/1 -> Sum19/2
  Sum10/1 -> Sum14/2
  roll/1 -> Sum22/2, Sum20/2, Sum6/2, Sum5/2, Sum1/2, Sum2/2
  pitch/1 -> Sum14/1, Sum24/1, Sum26/1, Sum13/1
  Sum13/1 -> front left/1
  Sum19/1 -> left/1
  Sum14/1 -> rear left/1
  Sum24/1 -> rear right/1
  Sum8/1 -> right/1
  Sum26/1 -> front rigth/1
  Constant/1 -> Sum3/2
  Sum3/1 -> Mux/2, Min/2  "to_max"
  Min/1 -> Gain1/1
  Mux/1 -> span-reserve/1
  Gain1/1 -> max-span/1
  Gain3/1 -> Mux/1, Min/1, Sum3/1, Sum22/1, Sum20/1, Sum6/1, Sum5/1, Sum2/1, Sum1/1

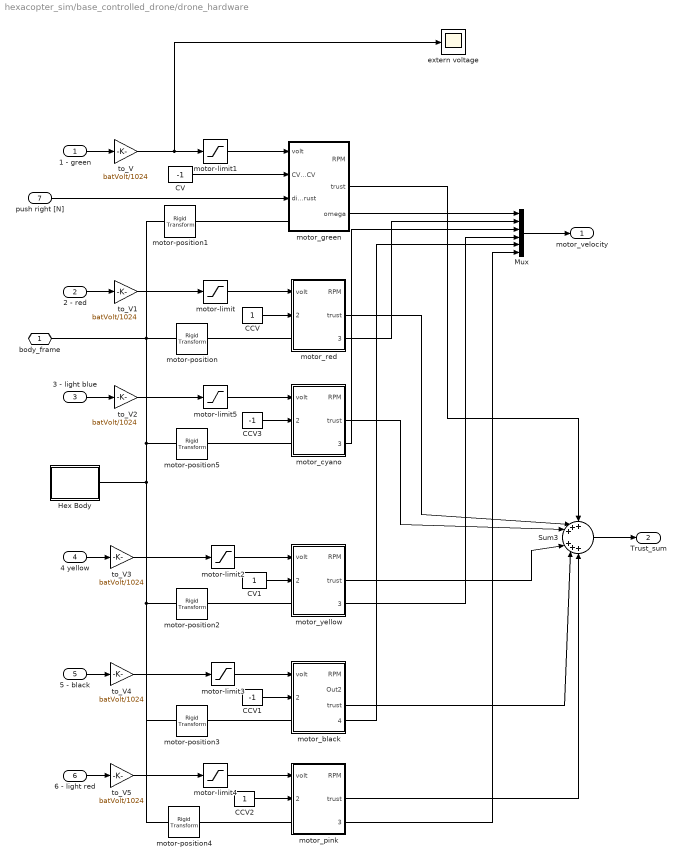
== system hexacopter_sim/base_controlled_drone/drone_hardware ==
  1 - green : Inport
  2 - red : Inport  Port=2
  3 - light blue : Inport  Port=3
  4 yellow : Inport  Port=4
  5 - black : Inport  Port=5
  6 - light red : Inport  Port=6
  push right [N] : Inport  Port=7
  CCV : Constant
  CCV1 : Constant  Value=-1
  CCV2 : Constant
  CCV3 : Constant  Value=-1
  CV : Constant  Value=-1
  CV1 : Constant
  Hex Body : Subsystem
      settings: PortSchema="{\"entries\":[{\"content\":{\"sides\":[{\"content\":{\"connectorIds\":[]},\"type\":\"ConnectorPlacement.EquallySpacedRectSide\",\"uuid\":\"01ed8a62-6d0e-429c-9fb0-ca702bbee18e\"},{\"content\":{\"connectorIds\":[],\"side\":\"RIGHT\"},\"type\":\"ConnectorPlacement.EquallySpacedRectSide\",\"uuid\":\"cdf1885d-1c5d-45e3-9572-3c603101c78e\"},{\"content\":{\"connectorIds\":[],\"side\":\"TOP\"},\"type\":\"ConnectorPlacement.EquallySpacedRectSide\",\"uuid\":\"9e81d776-774a-44d3-a154-58f7c6a5d82e\"},{\"content\":{\"connectorIds\":[\"RConn1\"],\"side\":\"BOTTOM\"},\"type\":\"ConnectorPlacement.EquallySpacedRectSide\",\"uuid\":\"9aef484f-1b98-4f15-b054-c09d0dce9b9e\"}]},\"type\":\"ConnectorPlacement.EquallySpacedConnector\",\"uuid\":\"2bac5469-8928-4e08-b1cb-20bc7858b0f9\"}],\"packageUris\":[\"http://schema.mathworks.com/mf0/Connector/19700101\"],\"version\":\"1.0\"}"
  Mux : Mux  Inputs=6
  Sum3 : Sum  Inputs=+++|+++
  extern voltage : Scope
  motor-limit{,1..5} (6 alike) : Saturate  UpperLimit=batVolt  LowerLimit=minimumMotorVolt
  motor-position : sm_lib/Frames and Transforms/Rigid Transform  TranslationMethod=Cylindrical  TranslationStandardOffset=0  TranslationStandardOffsetUnits=m  TranslationStandardAxis=+Z  TranslationCartesianOffset=[0 0.2 0.03]  TranslationCartesianOffsetUnits=m  TranslationROffset=arm_length  TranslationROffsetUnits=m  TranslationZOffset=0.03  TranslationZOffsetUnits=m  TranslationThetaOffset=-90  TranslationThetaOffsetUnits=deg  RotationMethod=StandardAxis  RotationAngleUnits=deg  RotationStandardAxis=+Y  RotationAngle=0.0  RotationArbitraryAxis=[0 0 1]  FollAlignAxisA=+X  BaseAlignAxisA=+Y  FollAlignAxisB=+Y  BaseAlignAxisB=+Z  RotationSequenceAxes=FollowerAxes  RotationSequence=XYX  RotationSequenceAngles=[0 0 0]  RotationSequenceAnglesUnits=deg  RotationMatrix=[1 0 0; 0 1 0; 0 0 1]  Quaternion=[1 0 0 0]
  motor-position1 : sm_lib/Frames and Transforms/Rigid Transform  TranslationMethod=Cylindrical  TranslationStandardOffset=0  TranslationStandardOffsetUnits=m  TranslationStandardAxis=+Z  TranslationCartesianOffset=[0 -0.2 0.03]  TranslationCartesianOffsetUnits=m  TranslationROffset=arm_length  TranslationROffsetUnits=m  TranslationZOffset=0.03  TranslationZOffsetUnits=m  TranslationThetaOffset=-30  TranslationThetaOffsetUnits=deg  RotationMethod=StandardAxis  RotationAngleUnits=deg  RotationStandardAxis=+Y  RotationAngle=0.0  RotationArbitraryAxis=[0 0 1]  FollAlignAxisA=+X  BaseAlignAxisA=+Y  FollAlignAxisB=+Y  BaseAlignAxisB=+Z  RotationSequenceAxes=FollowerAxes  RotationSequence=XYX  RotationSequenceAngles=[0 0 0]  RotationSequenceAnglesUnits=deg  RotationMatrix=[1 0 0; 0 1 0; 0 0 1]  Quaternion=[1 0 0 0]
  motor-position2 : sm_lib/Frames and Transforms/Rigid Transform  TranslationMethod=Cylindrical  TranslationStandardOffset=0  TranslationStandardOffsetUnits=m  TranslationStandardAxis=+Z  TranslationCartesianOffset=[0.2 0. 0.03]  TranslationCartesianOffsetUnits=m  TranslationROffset=arm_length  TranslationROffsetUnits=m  TranslationZOffset=0.03  TranslationZOffsetUnits=m  TranslationThetaOffset=+150  TranslationThetaOffsetUnits=deg  RotationMethod=StandardAxis  RotationAngleUnits=deg  RotationStandardAxis=+Y  RotationAngle=0.0  RotationArbitraryAxis=[0 0 1]  FollAlignAxisA=+X  BaseAlignAxisA=+Y  FollAlignAxisB=+Y  BaseAlignAxisB=+Z  RotationSequenceAxes=FollowerAxes  RotationSequence=XYX  RotationSequenceAngles=[0 0 0]  RotationSequenceAnglesUnits=deg  RotationMatrix=[1 0 0; 0 1 0; 0 0 1]  Quaternion=[1 0 0 0]
  motor-position3 : sm_lib/Frames and Transforms/Rigid Transform  TranslationMethod=Cylindrical  TranslationStandardOffset=0  TranslationStandardOffsetUnits=m  TranslationStandardAxis=+Z  TranslationCartesianOffset=[-0.2 0. 0.03]  TranslationCartesianOffsetUnits=m  TranslationROffset=arm_length  TranslationROffsetUnits=m  TranslationZOffset=0.03  TranslationZOffsetUnits=m  TranslationThetaOffset=90  TranslationThetaOffsetUnits=deg  RotationMethod=StandardAxis  RotationAngleUnits=deg  RotationStandardAxis=+Y  RotationAngle=0.0  RotationArbitraryAxis=[0 0 1]  FollAlignAxisA=+X  BaseAlignAxisA=+Y  FollAlignAxisB=+Y  BaseAlignAxisB=+Z  RotationSequenceAxes=FollowerAxes  RotationSequence=XYX  RotationSequenceAngles=[0 0 0]  RotationSequenceAnglesUnits=deg  RotationMatrix=[1 0 0; 0 1 0; 0 0 1]  Quaternion=[1 0 0 0]
  motor-position4 : sm_lib/Frames and Transforms/Rigid Transform  TranslationMethod=Cylindrical  TranslationStandardOffset=0  TranslationStandardOffsetUnits=m  TranslationStandardAxis=+Z  TranslationCartesianOffset=[-0.14 -0.14 0.03]  TranslationCartesianOffsetUnits=m  TranslationROffset=arm_length  TranslationROffsetUnits=m  TranslationZOffset=0.03  TranslationZOffsetUnits=m  TranslationThetaOffset=30  TranslationThetaOffsetUnits=deg  RotationMethod=StandardAxis  RotationAngleUnits=deg  RotationStandardAxis=+Y  RotationAngle=0.0  RotationArbitraryAxis=[0 0 1]  FollAlignAxisA=+X  BaseAlignAxisA=+Y  FollAlignAxisB=+Y  BaseAlignAxisB=+Z  RotationSequenceAxes=FollowerAxes  RotationSequence=XYX  RotationSequenceAngles=[0 0 0]  RotationSequenceAnglesUnits=deg  RotationMatrix=[1 0 0; 0 1 0; 0 0 1]  Quaternion=[1 0 0 0]
  motor-position5 : sm_lib/Frames and Transforms/Rigid Transform  TranslationMethod=Cylindrical  TranslationStandardOffset=0  TranslationStandardOffsetUnits=m  TranslationStandardAxis=+Z  TranslationCartesianOffset=[0.14 0.14 0.03]  TranslationCartesianOffsetUnits=m  TranslationROffset=arm_length  TranslationROffsetUnits=m  TranslationZOffset=0.03  TranslationZOffsetUnits=m  TranslationThetaOffset=-150  TranslationThetaOffsetUnits=deg  RotationMethod=StandardAxis  RotationAngleUnits=deg  RotationStandardAxis=+Y  RotationAngle=0.0  RotationArbitraryAxis=[0 0 1]  FollAlignAxisA=+X  BaseAlignAxisA=+Y  FollAlignAxisB=+Y  BaseAlignAxisB=+Z  RotationSequenceAxes=FollowerAxes  RotationSequence=XYX  RotationSequenceAngles=[0 0 0]  RotationSequenceAnglesUnits=deg  RotationMatrix=[1 0 0; 0 1 0; 0 0 1]  Quaternion=[1 0 0 0]
  motor_black : Subsystem
  motor_cyano : Subsystem
  motor_green : Subsystem
  motor_pink : Subsystem
  motor_red : Subsystem
  motor_yellow : Subsystem
  to_V{,1..5} (6 alike) : Gain  Gain=batVolt/1024
  body_frame : PMIOPort  Side=Left
  motor_velocity : Outport  VectorParamsAs1DForOutWhenUnconnected=off
  Trust_sum : Outport  Port=2  VectorParamsAs1DForOutWhenUnconnected=off
  wires:
  1 - green/1 -> to_V/1
  push right [N]/1 -> motor_green/3(disturb_trust)
  motor_green/2(trust) -> Sum3/1
  motor_red/2(trust) -> Sum3/2
  CV/1 -> motor_green/2(CV_CCV)
  motor-limit1/1 -> motor_green/1(volt)
  CCV/1 -> motor_red/2(CV_CCV)
  Mux/1 -> motor_velocity/1
  Sum3/1 -> Trust_sum/1
  2 - red/1 -> to_V1/1
  motor-limit/1 -> motor_red/1(volt)
  4 yellow/1 -> to_V3/1
  motor-limit2/1 -> motor_yellow/1(volt)
  5 - black/1 -> to_V4/1
  motor-limit3/1 -> motor_black/1(volt)
  CCV1/1 -> motor_black/2(CV_CCV)
  CV1/1 -> motor_yellow/2(CV_CCV)
  motor_yellow/2(trust) -> Sum3/4
  motor_pink/2(trust) -> Sum3/6
  6 - light red/1 -> to_V5/1
  motor-limit4/1 -> motor_pink/1(volt)
  CCV2/1 -> motor_pink/2(CV_CCV)
  3 - light blue/1 -> to_V2/1
  motor-limit5/1 -> motor_cyano/1(volt)
  CCV3/1 -> motor_cyano/2(CV_CCV)
  motor_cyano/2(trust) -> Sum3/3
  motor_green/3(omega) -> Mux/1
  motor_red/3(omega) -> Mux/2
  motor_cyano/3(omega) -> Mux/3
  motor_yellow/3(omega) -> Mux/4
  motor_black/4(omega) -> Mux/5
  motor_pink/3(omega) -> Mux/6
  to_V/1 -> extern voltage/1, motor-limit1/1
  to_V1/1 -> motor-limit/1
  to_V2/1 -> motor-limit5/1
  to_V3/1 -> motor-limit2/1
  to_V4/1 -> motor-limit3/1
  to_V5/1 -> motor-limit4/1
  motor_black/3(trust) -> Sum3/5
  connections:
  motor-position5/LConn1 -- motor-position3/LConn1 -- motor-position4/LConn1 -- motor-position2/LConn1 -- Hex Body/RConn1 -- body_frame/RConn1 -- motor-position/LConn1 -- motor-position1/LConn1
  motor-position1/RConn1 -- motor_green/LConn1
  motor_red/LConn1 -- motor-position/RConn1
  motor_yellow/LConn1 -- motor-position2/RConn1
  motor_black/LConn1 -- motor-position3/RConn1
  motor_pink/LConn1 -- motor-position4/RConn1
  motor_cyano/LConn1 -- motor-position5/RConn1

== system hexacopter_sim/base_controlled_drone/height complement filter ==
  z-pos : Inport
  z-acc : Inport  Port=2
  Gain : Gain  Gain=h_tau
  Mux1 : Mux  Inputs=5
  Sum2 : Sum  Inputs=|++
  Transfer Fcn2 : TransferFcn  Denominator=[h_tau 1]
  Transfer Fcn4 : TransferFcn  Numerator=[h_tau*h_beta]  Denominator=[h_tau*h_beta 1]
  filtered height1 : Scope
  1. order filt : Outport
  height velocity : Outport  Port=2
  wires:
  Gain/1 -> Sum2/2, Mux1/3  "1. order filt_acc"
  z-pos/1 -> Mux1/4, Mux1/1, Sum2/1  "pressure_height"
  Transfer Fcn4/1 -> height velocity/1, Mux1/5, Gain/1  "height vel"
  Sum2/1 -> Transfer Fcn2/1
  z-acc/1 -> Transfer Fcn4/1
  Mux1/1 -> filtered height1/1
  Transfer Fcn2/1 -> Mux1/2, 1. order filt/1  "1. order filt_acc"

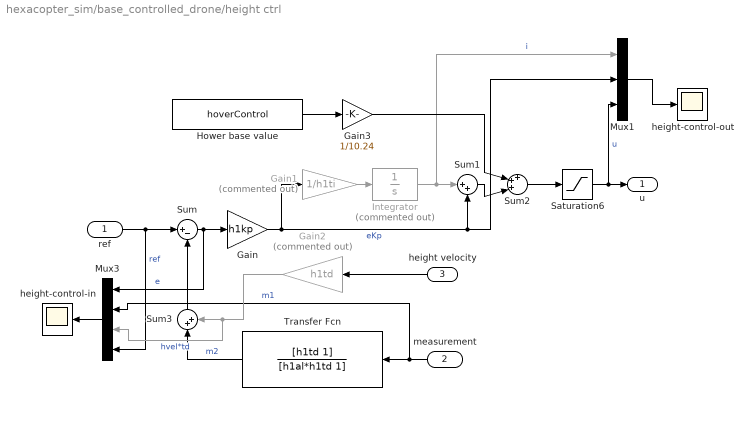
== system hexacopter_sim/base_controlled_drone/height ctrl ==
  ref : Inport
  measurement : Inport  Port=2
  height velocity : Inport  Port=3
  Gain : Gain  Gain=h1kp
  Gain1 : Gain  Commented=on  Gain=1/h1ti
  Gain2 : Gain  Commented=on  Gain=h1td
  Gain3 : Gain  Gain=1/10.24
  Hower base value : Constant  Value=hoverControl
  Integrator : Integrator  Commented=on  InitialCondition=minimumMotorVolt  LimitOutput=on  UpperSaturationLimit=1000  LowerSaturationLimit=-1000
  Mux1 : Mux  Inputs=3
  Mux3 : Mux
  Saturation6 : Saturate  UpperLimit=1024*0.95  LowerLimit=1
  Sum : Sum  Inputs=|+-
  Sum1 : Sum  Inputs=|++
  Sum2 : Sum  Inputs=+++|
  Sum3 : Sum  Inputs=|++
  Transfer Fcn : TransferFcn  Numerator=[h1td 1]  Denominator=[h1al*h1td 1]
  height-control-in : Scope
  height-control-out : Scope
  u : Outport  VectorParamsAs1DForOutWhenUnconnected=off
  wires:
  ref/1 -> Mux3/4, Sum/1  "ref"
  measurement/1 -> Mux3/2, Transfer Fcn/1  "m1"
  Sum/1 -> Mux3/1, Gain/1  "e"
  Integrator/1 -> Mux1/1, Sum1/1  "i"
  Gain1/1 -> Integrator/1
  Mux3/1 -> height-control-in/1
  Saturation6/1 -> Mux1/3, u/1  "u"
  Gain/1 -> Gain1/1, Sum1/2, Mux1/2  "eKp"
  Mux1/1 -> height-control-out/1
  Sum2/1 -> Saturation6/1
  Sum1/1 -> Sum2/3
  Transfer Fcn/1 -> Sum3/1  "m2"
  height velocity/1 -> Gain2/1
  Gain2/1 -> Mux3/3, Sum3/2  "hvel*td"
  Hower base value/1 -> Gain3/1
  Sum3/1 -> Sum/2
  Gain3/1 -> Sum2/2

== system hexacopter_sim/base_controlled_drone/height_vel ==
  ref : Inport
  measurement : Inport  Port=2
  Gain : Gain  Gain=h1vkp
  Gain1 : Gain  Gain=1/h1vti
  Integrator : Integrator  LimitOutput=on  UpperSaturationLimit=1024*0.10  LowerSaturationLimit=-1024*0.10
  Scope{,1..3} (4 alike) : Scope
  Sum : Sum  Inputs=|+-
  Sum1 : Sum  Inputs=|++
  Transfer Fcn : TransferFcn  Numerator=[h1vtd 1]  Denominator=[h1val*h1vtd 1]
  u : Outport  VectorParamsAs1DForOutWhenUnconnected=off
  wires:
  ref/1 -> Scope2/1, Sum/1
  measurement/1 -> Transfer Fcn/1
  Transfer Fcn/1 -> Scope3/1, Sum/2
  Sum/1 -> Scope1/1, Gain/1
  Sum1/1 -> Scope/1, u/1
  Integrator/1 -> Sum1/1
  Gain/1 -> Sum1/2, Gain1/1
  Gain1/1 -> Integrator/1

== system hexacopter_sim/base_controlled_drone/pitch ctrl ==
  ref : Inport
  measurement : Inport  Port=2
  Gain : Gain  Gain=pakp
  Gain1 : Gain  Commented=on  Gain=1/pati
  Integrator : Integrator  Commented=on  InitialCondition=hoverVoltage  LimitOutput=on  UpperSaturationLimit=batVolt  LowerSaturationLimit=-batVolt
  Sum : Sum  Inputs=|+-
  Sum1 : Sum  Inputs=|++
  Transfer Fcn : TransferFcn  Numerator=[patd 1]  Denominator=[paal*patd 1]
  u : Outport  VectorParamsAs1DForOutWhenUnconnected=off
  wires:
  Gain1/1 -> Integrator/1
  Gain/1 -> Sum1/2, Gain1/1
  Integrator/1 -> Sum1/1
  Sum1/1 -> u/1
  Sum/1 -> Gain/1
  Transfer Fcn/1 -> Sum/2
  measurement/1 -> Transfer Fcn/1
  ref/1 -> Sum/1

== system hexacopter_sim/base_controlled_drone/pitch vel ctrl ==
  ref : Inport
  measurement : Inport  Port=2
  Gain : Gain  Gain=pkp
  Gain1 : Gain  Commented=on  Gain=1/pti
  Integrator : Integrator  Commented=on  InitialCondition=hoverVoltage  LimitOutput=on  UpperSaturationLimit=batVolt  LowerSaturationLimit=-batVolt
  Sum : Sum  Inputs=|+-
  Sum1 : Sum  Inputs=|++
  Transfer Fcn : TransferFcn  Numerator=[ptd 1]  Denominator=[pal*ptd 1]
  Transfer Fcn1 : TransferFcn  Commented=through  Denominator=[0.02 1]
  u : Outport  VectorParamsAs1DForOutWhenUnconnected=off
  wires:
  ref/1 -> Sum/1
  measurement/1 -> Transfer Fcn/1
  Transfer Fcn/1 -> Sum/2
  Sum/1 -> Gain/1
  Sum1/1 -> Transfer Fcn1/1
  Integrator/1 -> Sum1/1
  Gain/1 -> Gain1/1, Sum1/2
  Gain1/1 -> Integrator/1
  Transfer Fcn1/1 -> u/1
